simulink model "test_direct"  (R2024a)
(part 32 of 35)

  "IW{4,3}(6,:)'" : Constant  Value=[-0.1446227260697748040474408526279148645699024200439453125;-0.2535207694767447339501131864381022751331329345703125;0.01232111902921316330672407701740667107515037059783935546875;-0.195255356855180917108327776077203452587127685546875;-0.0176116564122183703877677629634490585885941982269287109375;-0.2307620350490153515732316691355663351714611053466796875;0.08613137628681850899159400114513118751347064971923828125;-0.1475666915697550762853751393777201883494853973388671875;-0.1398125565568799633098251433693803846836090087890625;-0.00553863677515696421760349466012485208921134471893310546875;-0.1766227926639023504407077780342660844326019287109375;-0.025502761693635779549627073947704047895967960357666015625;0.179621033504632821031776757081388495862483978271484375;0.1826757008565532414134935379479429684579372406005859375;-0.01291552840292176616843189407290992676280438899993896484375;0.26313281165259494454033983856788836419582366943359375;0.131071308290465093904231252963654696941375732421875;0.27681360897790308062127451194101013243198394775390625;-0.136538807870576761605008186961640603840351104736328125;0.145222911984573876953419357960228808224201202392578125;0.0974186206438350243974610975783434696495532989501953125;0.041872513522693673160279814737805281765758991241455078125;0.0809424357153154805377681668687728233635425567626953125;-0.08543750561650413632985845424627768807113170623779296875;-0.213276602632264944414686169693595729768276214599609375;-0.0202950036140331670220238180490923696197569370269775390625;-0.2265254594046355596237418694727239198982715606689453125;-0.2282716871019460913583287720030057244002819061279296875;-0.2747579782172453466415618095197714865207672119140625;0.271964132672625924502796124215819872915744781494140625;-0.0661299794756544379037421776956762187182903289794921875;-0.1958504023465361398859130304117570631206035614013671875;-0.25524857590640548377081131548038683831691741943359375;0.15762991974972262454457450076006352901458740234375;-0.050643939147725254568133124166706693358719348907470703125;-0.04797070265166240854437518237318727187812328338623046875;0.2755110868022481174222093613934703171253204345703125;-0.241538803893189213400916059981682337820529937744140625;-0.2693164235740115319828191786655224859714508056640625;-0.08983963142694013914724138203382608480751514434814453125;0.11632586875825122463279370776945143006742000579833984375;0.2221370724402033924871346926011028699576854705810546875;0.312263129526412275271951557442662306129932403564453125;0.1763043373643742028900049945150385610759258270263671875;0.00472671747490137524050357598071059328503906726837158203125;0.1353418593240807432653838304759119637310504913330078125;-0.347154273516572520197343010295298881828784942626953125;0.000902754956261455081441280601239895986509509384632110595703125;0.23886841550304416248451389037654735147953033447265625;0.05403647704435020349134077832786715589463710784912109375;0.253788690960465412871371881919912993907928466796875;0.1193284933714482687339142330529284663498401641845703125;0.26903689147685250215857877265079878270626068115234375;-0.010986001921949241355580539902803138829767704010009765625;-0.268857961659322575176389591433689929544925689697265625;0.0627120691048583811522121322923339903354644775390625;-0.127268307829933202679484338659676723182201385498046875;-0.147990099867200519678789305544341914355754852294921875;0.1618899914170077447561624239824595861136913299560546875;0.321930080837258103532150244063814170658588409423828125]
      mask Display: e = 0.06;c1 = [120 150 230]/255;c2 = ([120 150 230]+0)/383;c3 = ([120 150 230]+128)/383;patch([0 1 1 0],[0 0 1 1],c1);patch([0 1 1 1-e 1-e 0+e],[0 0 1 1-e 0+e 0+e],c2);patch([0 0 1 1-e 0+e 0+e],[0 1 1 1-e 1-e 0+e],c3);plot([0 1 1 0 0],[0 0 1 1 0]);disp('weights');
  "IW{4,3}(7,:)'" : Constant  Value=[0.2289221792326882887191885629363241605460643768310546875;0.3119956532937215865075586407328955829143524169921875;0.07724042267836768449473794362347689457237720489501953125;-0.1665292171214766969722376188656198792159557342529296875;0.06456819592207017899365695257074548862874507904052734375;-0.30235772642395886133925841932068578898906707763671875;0.1967369766784285156635547764381044544279575347900390625;0.1689164759704222251723848557958262972533702850341796875;0.162531028279926770263585922293714247643947601318359375;-0.3011510237839398751447106405976228415966033935546875;0.11620641226252929889550813413734431378543376922607421875;-0.281442609407358046436087306574336253106594085693359375;-0.041353244682499575024525739763703313656151294708251953125;-0.121516768306712374947409216474625281989574432373046875;0.093996035776526210003822825456154532730579376220703125;0.035008805502344524096525191225737216882407665252685546875;-0.02648565784088664776252386445776210166513919830322265625;0.3007680707458677549226422343053855001926422119140625;0.0778641152526692026381027744719176553189754486083984375;0.1375528560683864920388685959551366977393627166748046875;-0.1687452370705504467451874006655998528003692626953125;-0.1771988365206792759298792816480272449553012847900390625;-0.315828222276993975103920320179895497858524322509765625;0.1474140604552382216585471041980781592428684234619140625;0.007784432653196713715326726656940081738866865634918212890625;-0.0437125695684012216535307970843859948217868804931640625;-0.162612629683519249734757750047720037400722503662109375;-0.23504079282243217630110621030326001346111297607421875;0.31236358902008676263761799418716691434383392333984375;0.32404192989106028743861998009379021823406219482421875;-0.04202990397551997769909348789951764047145843505859375;0.238725479452904509880539762889384292066097259521484375;0.2517535838714934914861487413872964680194854736328125;-0.27404887557243962081798827057355083525180816650390625;0.0207631966962754134498059244151590974070131778717041015625;-0.255191567857939782815179796671145595610141754150390625;-0.27924773068630714956128713311045430600643157958984375;-0.070636518954219129629024109817692078649997711181640625;-0.000460014527161740384431087846905938931740820407867431640625;0.1367885574957196370693424114506342448294162750244140625;0.1519055638686676867887825892466935329139232635498046875;0.14815607894696836144277085622888989746570587158203125;0.265985233461738468374591093379422090947628021240234375;0.050259191345343234846865243525826372206211090087890625;-0.11462677289128149482611007670129765756428241729736328125;-0.1547603558767412235130933595428359694778919219970703125;0.301182427802490104706834017633809708058834075927734375;-0.074355957455443100201364359236322343349456787109375;0.0266149070353163298696674843313303426839411258697509765625;-0.225233741194319880829510793773806653916835784912109375;-0.245534495354167103808862293590209446847438812255859375;0.11902702333813854063127024573987000621855258941650390625;0.11515347999788803912135648488401784561574459075927734375;-0.2269011222377796122007254098207340575754642486572265625;0.21663359331567288990072484011761844158172607421875;0.144143426337712210472119522819411940872669219970703125;0.28604930059216837623381479716044850647449493408203125;-0.3554517488762976018534800459747202694416046142578125;-0.07545651379027897009965641927919932641088962554931640625;-0.050995757215796889971759497939274297095835208892822265625]
      mask Display: e = 0.06;c1 = [120 150 230]/255;c2 = ([120 150 230]+0)/383;c3 = ([120 150 230]+128)/383;patch([0 1 1 0],[0 0 1 1],c1);patch([0 1 1 1-e 1-e 0+e],[0 0 1 1-e 0+e 0+e],c2);patch([0 0 1 1-e 0+e 0+e],[0 1 1 1-e 1-e 0+e],c3);plot([0 1 1 0 0],[0 0 1 1 0]);disp('weights');
  "IW{4,3}(8,:)'" : Constant  Value=[0.1078351843868104731338775081894709728658199310302734375;0.1864376580391729765207031732643372379243373870849609375;0.222692427561942463132282910009962506592273712158203125;0.2484574185053898542907546698188525624573230743408203125;-0.1396405295594020101734855643371702171862125396728515625;0.0218708959701903772609998810594333917833864688873291015625;0.2147510481991358466391517367810592986643314361572265625;0.137404881875626661003053641252336092293262481689453125;0.08536956260653795480752847879557521082460880279541015625;-0.0161509590905200284272069666258175857365131378173828125;0.253381779373638871266649630342726595699787139892578125;0.358755636755657747460901418889989145100116729736328125;-0.22473880489791853154457612617989070713520050048828125;-0.2854522236169090287916105808108113706111907958984375;-0.061627460324472548014451689368797815404832363128662109375;0.224082124747383815144274876729468815028667449951171875;-0.258386245491298460752460641742800362408161163330078125;0.12446319745409444024186740307413856498897075653076171875;0.1854709573317227244704241684303269721567630767822265625;0.1132690436769869524180620601327973417937755584716796875;-0.297886886497514435934164112040889449417591094970703125;0.2067076799767223749260125487126060761511325836181640625;0.21924415347157755196150219489936716854572296142578125;-0.44075382417526665079776648781262338161468505859375;0.0467682082280729549683684354022261686623096466064453125;-0.258991068241769095692461633007042109966278076171875;-0.0899096615289569911499967247436870820820331573486328125;0.17392231152049186793107082849019207060337066650390625;0.13843030299286229745092668963479809463024139404296875;0.301596457539933859859360154587193392217159271240234375;0.04763810315894816127535449368224362842738628387451171875;-0.00048790694574566318038322254579952641506679356098175048828125;-0.11336618048125964020034217583088320679962635040283203125;-0.034543869085566468457582089968127547763288021087646484375;-0.07306197035299359654469952829458634369075298309326171875;0.23262052363997043347154658476938493549823760986328125;-0.0232042088426238878040575031036496511660516262054443359375;0.276321286471199190071246221123146824538707733154296875;-0.277980384596168084154754751580185256898403167724609375;0.299711183824943161457809992498368956148624420166015625;0.0315604595426603184993297190885641612112522125244140625;0.298470717978130739567177442950196564197540283203125;-0.168088831833297813744820814463309943675994873046875;0.0782001968165516869735398586271912790834903717041015625;0.07105307175157872523474367199014523066580295562744140625;0.240790077827006399058262786638806574046611785888671875;0.1695099595809218262498774265623069368302822113037109375;-0.1920518850777122865647328353588818572461605072021484375;0.1255596935081750575857739704588311724364757537841796875;0.235863928290519719865869774366728961467742919921875;0.07607933828919728747042228178543155081570148468017578125;-0.2046838608270919179776825558292330242693424224853515625;-0.069137488624790688351851031256956048309803009033203125;0.1308228814165624254162167972026509232819080352783203125;0.276561829811876602747133802040480077266693115234375;-0.206893520137229725008864988922141492366790771484375;-0.142753587117182834109740952044376172125339508056640625;0.1981888971831225754183236631433828733861446380615234375;0.14444267200677263218722146120853722095489501953125;-0.040463678308624677348870335436004097573459148406982421875]
      mask Display: e = 0.06;c1 = [120 150 230]/255;c2 = ([120 150 230]+0)/383;c3 = ([120 150 230]+128)/383;patch([0 1 1 0],[0 0 1 1],c1);patch([0 1 1 1-e 1-e 0+e],[0 0 1 1-e 0+e 0+e],c2);patch([0 0 1 1-e 0+e 0+e],[0 1 1 1-e 1-e 0+e],c3);plot([0 1 1 0 0],[0 0 1 1 0]);disp('weights');
  "IW{4,3}(9,:)'" : Constant  Value=[0.024391016990708148937105903542033047415316104888916015625;-0.0922419336882071838612517922229017131030559539794921875;0.2610178043953812476729581248946487903594970703125;-0.0031092423320425804054989438185430117300711572170257568359375;-0.08456363520575384262745188834742293693125247955322265625;0.034863543566850112298549646538958768360316753387451171875;0.10489127078132480519467861768134753219783306121826171875;0.2112649033662876429939814215686055831611156463623046875;-0.08028846966605850121734277990981354378163814544677734375;0.2406552349892890629856623263549408875405788421630859375;0.09025963910876122486826034219120629131793975830078125;0.044676408936308122099578810093589709140360355377197265625;0.2361000840904136366393828438958735205233097076416015625;0.260715562546214585371018301884760148823261260986328125;0.1588054433831249667719021090306341648101806640625;-0.29360419404964088752052475683740340173244476318359375;0.056829196108893094419034497377651860006153583526611328125;0.109923340167149052870598779918509535491466522216796875;0.0703697020926560001807814614949165843427181243896484375;-0.245313812713407408683252697301213629543781280517578125;-0.2992407965870815811371130621409974992275238037109375;0.10908561804925233362784098289921530522406101226806640625;-0.32159333423413005714763812648016028106212615966796875;-0.3233709253851824172443230054341256618499755859375;-0.32703025244063665954996622531325556337833404541015625;0.1268016484898610574116872840022551827132701873779296875;0.29417701972544241240115070468164049088954925537109375;-0.2395906388579759072054997659506625495851039886474609375;0.2061606018933385409130920606912695802748203277587890625;0.2277674969607056121301269513423903845250606536865234375;-0.22009105103668147318529690892319194972515106201171875;0.07478323862371853703034929594650748185813426971435546875;0.1690603118789672787425359956614556722342967987060546875;0.056733607128887086901158909313380718231201171875;0.149314514854280322442292572304722853004932403564453125;0.2677532950739998085509796510450541973114013671875;-0.2402854326691058750586904579904512502253055572509765625;-0.274665973904204718802901652452419511973857879638671875;-0.0720651556117201386175707966685877181589603424072265625;-0.267868382192499698835064236845937557518482208251953125;-0.2354425302245911344467543813152587972581386566162109375;-0.266667813995020097639354617058415897190570831298828125;-0.0463160235831618638524531661460059694945812225341796875;0.1506242400717603679982659059533034451305866241455078125;0.07294388497646649149874775730495457537472248077392578125;0.052719940543337819038871572274729260243475437164306640625;-0.2193790501091265332522795006298110820353031158447265625;-0.00195057812244301006197877423886666292673908174037933349609375;0.13011900811869636651607606836478225886821746826171875;0.270790108694598685712406904713134281337261199951171875;0.18839902311572787052540434160619042813777923583984375;-0.087407536202535551783654454993666149675846099853515625;-0.1972482903530723696849946691145305521786212921142578125;-0.1745780971902311795584950004922575317323207855224609375;-0.0130985572525647957220495953833960811607539653778076171875;-0.2464905123848703250022396105123334564268589019775390625;-0.165283747715149254009503465567831881344318389892578125;-0.259143413148147094826612146789557300508022308349609375;0.195683676278246176938324651928269304335117340087890625;0.1491305033088377030026094871573150157928466796875]
      mask Display: e = 0.06;c1 = [120 150 230]/255;c2 = ([120 150 230]+0)/383;c3 = ([120 150 230]+128)/383;patch([0 1 1 0],[0 0 1 1],c1);patch([0 1 1 1-e 1-e 0+e],[0 0 1 1-e 0+e 0+e],c2);patch([0 0 1 1-e 0+e 0+e],[0 1 1 1-e 1-e 0+e],c3);plot([0 1 1 0 0],[0 0 1 1 0]);disp('weights');
  Mux : Mux  Inputs=40
      mask Display: e = 0.06;c1 = [120 150 230]/255;c2 = ([120 150 230]+0)/383;c3 = ([120 150 230]+128)/383;patch([0 1 1 0],[0 0 1 1],c1);patch([0 1 1 1-e 1-e 0+e],[0 0 1 1-e 0+e 0+e],c2);patch([0 0 1 1-e 0+e 0+e],[0 1 1 1-e 1-e 0+e],c3);plot([0 1 1 0 0],[0 0 1 1 0]);disp('Mux');
  dotprod{1..40} (40 alike) : neural/Weight Functions/dotprod
  "lz{4,3}" : Outport
      mask Display: e = 0.06;c1 = [120 230 180]/255;c2 = ([120 230 180]+0)/(256+128);c3 = ([120 230 180]+128)/(256+128);patch([0 1 1 0],[0 0 1 1],c1);patch([0 1 1 1-e 1-e 0+e],[0 0 1 1-e 0+e 0+e],c2);patch([0 0 1 1-e 0+e 0+e],[0 1 1 1-e 1-e 0+e],c3);plot([0 1 1 0 0],[0 0 1 1 0]);
  wires:
  "IW{4,3}(1,:)'"/1 -> dotprod1/1
  "ad{4,3}"/1 -> dotprod1/2, dotprod2/2, dotprod3/2, dotprod4/2, dotprod5/2, dotprod6/2, dotprod7/2, dotprod8/2, dotprod9/2, dotprod10/2, dotprod11/2, dotprod12/2, dotprod13/2, dotprod14/2, dotprod15/2, dotprod16/2, dotprod17/2, dotprod18/2, dotprod19/2, dotprod20/2, dotprod21/2, dotprod22/2, dotprod23/2, dotprod24/2, dotprod25/2, dotprod26/2, dotprod27/2, dotprod28/2, dotprod29/2, dotprod30/2, dotprod31/2, dotprod32/2, dotprod33/2, dotprod34/2, dotprod35/2, dotprod36/2, dotprod37/2, dotprod38/2, dotprod39/2, dotprod40/2
  dotprod1/1 -> Mux/1
  "IW{4,3}(2,:)'"/1 -> dotprod2/1
  dotprod2/1 -> Mux/2
  "IW{4,3}(3,:)'"/1 -> dotprod3/1
  dotprod3/1 -> Mux/3
  "IW{4,3}(4,:)'"/1 -> dotprod4/1
  dotprod4/1 -> Mux/4
  "IW{4,3}(5,:)'"/1 -> dotprod5/1
  dotprod5/1 -> Mux/5
  "IW{4,3}(6,:)'"/1 -> dotprod6/1
  dotprod6/1 -> Mux/6
  "IW{4,3}(7,:)'"/1 -> dotprod7/1
  dotprod7/1 -> Mux/7
  "IW{4,3}(8,:)'"/1 -> dotprod8/1
  dotprod8/1 -> Mux/8
  "IW{4,3}(9,:)'"/1 -> dotprod9/1
  dotprod9/1 -> Mux/9
  "IW{4,3}(10,:)'"/1 -> dotprod10/1
  dotprod10/1 -> Mux/10
  "IW{4,3}(11,:)'"/1 -> dotprod11/1
  dotprod11/1 -> Mux/11
  "IW{4,3}(12,:)'"/1 -> dotprod12/1
  dotprod12/1 -> Mux/12
  "IW{4,3}(13,:)'"/1 -> dotprod13/1
  dotprod13/1 -> Mux/13
  "IW{4,3}(14,:)'"/1 -> dotprod14/1
  dotprod14/1 -> Mux/14
  "IW{4,3}(15,:)'"/1 -> dotprod15/1
  dotprod15/1 -> Mux/15
  "IW{4,3}(16,:)'"/1 -> dotprod16/1
  dotprod16/1 -> Mux/16
  "IW{4,3}(17,:)'"/1 -> dotprod17/1
  dotprod17/1 -> Mux/17
  "IW{4,3}(18,:)'"/1 -> dotprod18/1
  dotprod18/1 -> Mux/18
  "IW{4,3}(19,:)'"/1 -> dotprod19/1
  dotprod19/1 -> Mux/19
  "IW{4,3}(20,:)'"/1 -> dotprod20/1
  dotprod20/1 -> Mux/20
  "IW{4,3}(21,:)'"/1 -> dotprod21/1
  dotprod21/1 -> Mux/21
  "IW{4,3}(22,:)'"/1 -> dotprod22/1
  dotprod22/1 -> Mux/22
  "IW{4,3}(23,:)'"/1 -> dotprod23/1
  dotprod23/1 -> Mux/23
  "IW{4,3}(24,:)'"/1 -> dotprod24/1
  dotprod24/1 -> Mux/24
  "IW{4,3}(25,:)'"/1 -> dotprod25/1
  dotprod25/1 -> Mux/25
  "IW{4,3}(26,:)'"/1 -> dotprod26/1
  dotprod26/1 -> Mux/26
  "IW{4,3}(27,:)'"/1 -> dotprod27/1
  dotprod27/1 -> Mux/27
  "IW{4,3}(28,:)'"/1 -> dotprod28/1
  dotprod28/1 -> Mux/28
  "IW{4,3}(29,:)'"/1 -> dotprod29/1
  dotprod29/1 -> Mux/29
  "IW{4,3}(30,:)'"/1 -> dotprod30/1
  dotprod30/1 -> Mux/30
  "IW{4,3}(31,:)'"/1 -> dotprod31/1
  dotprod31/1 -> Mux/31
  "IW{4,3}(32,:)'"/1 -> dotprod32/1
  dotprod32/1 -> Mux/32
  "IW{4,3}(33,:)'"/1 -> dotprod33/1
  dotprod33/1 -> Mux/33
  "IW{4,3}(34,:)'"/1 -> dotprod34/1
  dotprod34/1 -> Mux/34
  "IW{4,3}(35,:)'"/1 -> dotprod35/1
  dotprod35/1 -> Mux/35
  "IW{4,3}(36,:)'"/1 -> dotprod36/1
  dotprod36/1 -> Mux/36
  "IW{4,3}(37,:)'"/1 -> dotprod37/1
  dotprod37/1 -> Mux/37
  "IW{4,3}(38,:)'"/1 -> dotprod38/1
  dotprod38/1 -> Mux/38
  "IW{4,3}(39,:)'"/1 -> dotprod39/1
  dotprod39/1 -> Mux/39
  "IW{4,3}(40,:)'"/1 -> dotprod40/1
  dotprod40/1 -> Mux/40
  Mux/1 -> "lz{4,3}"/1
